simulink model "c"  (R2020a)
settings: Solver=VariableStepAuto  StartTime=0.0  StopTime=50  RelTol=1e-3
settings Model: Creator=hp  LastModifiedBy=hp

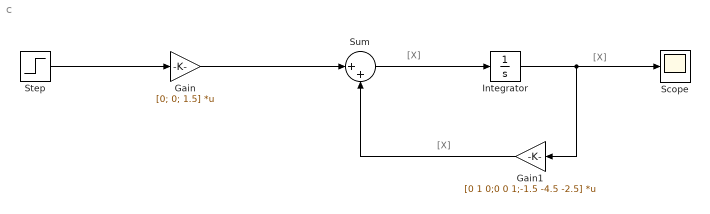
== system c ==
  note: [X]
  note: [X]
  note: [X]
  Gain : Gain  Gain=[0; 0; 1.5]  Multiplication=Matrix(K*u)
  Gain1 : Gain  Gain=[0 1 0;0 0 1;-1.5 -4.5 -2.5]  Multiplication=Matrix(K*u)
  Integrator : Integrator
  Scope : Scope
  Step : Step  SampleTime=0
  Sum : Sum  Inputs=|++
  wires:
  Gain1/1 -> Sum/2
  Gain/1 -> Sum/1
  Step/1 -> Gain/1
  Integrator/1 -> Gain1/1, Scope/1
  Sum/1 -> Integrator/1
